simulink model "SubHubmagnet"  (R2020b)
settings: Solver=FixedStepAuto  StartTime=0.0  StopTime=10.0  FixedStep=0.001  RelTol=1e-3
settings Model: Creator=kaebi  LastModifiedBy=kaebi
settings ConfigComp: PLC_TargetIDE=twincat3

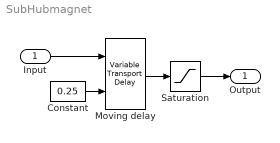
== system SubHubmagnet ==
  Input : Inport
  Constant : Constant  Value=0.25
  Moving delay : VariableTransportDelay  MaximumDelay=10
  Saturation : Saturate  UpperLimit=1  LowerLimit=0
  Output : Outport
  wires:
  Constant/1 -> Moving delay/2
  Input/1 -> Moving delay/1
  Moving delay/1 -> Saturation/1
  Saturation/1 -> Output/1
